simulink model "MotorSimlab4"  (R2015b)
settings: Solver=ode4  StartTime=0.0  StopTime=10  FixedStep=0.001  RelTol=1e-3
values from neighbouring files (symbols this model uses):
  Beq = BeqHigh    (= 0.015)    [transferfunctionlab4.m]
  Jeq = JeqPaper    (= 0.00213)    [transferfunctionlab4.m]
  Ka = KaHigh    (= 3420.59016393)    [transferfunctionlab4.m]
  Kb = KbHigh    (= 0.5376)    [transferfunctionlab4.m]
  Kg = KgHigh    (= 70)    [transferfunctionlab4.m]
  Rm = 2.6    [transferfunctionlab4.m]
undefined symbols (not defined in the file or in its folder): HIL, qc_get_step_size
libraries: quarc_library x4
settings Model: SimulationMode=external  ExtModeTrigDuration=10000  Creator=dilsizk  LastModifiedBy=dilsizk
settings SolverCC: PositivePriorityOrder=on
settings RTWCC: SystemTargetFile=quarc_win64.tlc  TemplateMakefile=quarc_default_tmf  Description=QUARC Win64 Target
settings STFCustomTargetCC: TargetPreCompLibLocation=C:\ProgramData\QUARC\lib\2015b\win64\release  GeneratePreprocessorConditionals=Use local settings  CPPClassGenCompliant=off
settings GRTTargetCC: TargetPreCompLibLocation=C:\ProgramData\QUARC\lib\2015b\win64\release  ParMdlRefBuildCompliant=off  CompOptLevelCompliant=off  CombineOutputUpdateFcns=off  MatFileLogging=off  CPPClassGenCompliant=off  GRTInterface=on  UseToolchainInfoCompliant=off  ExtMode=on  ExtModeMexFile=quarc_comm

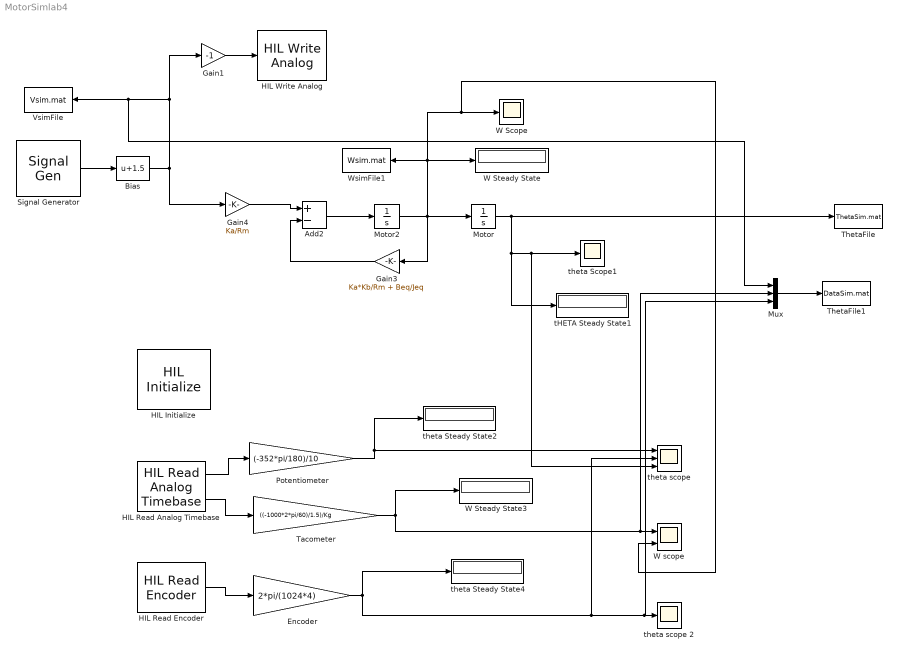
== system MotorSimlab4 ==
  Add2 : Sum  Inputs=+-
  Bias : Bias  Bias=1.5
  Encoder : Gain  Gain=2*pi/(1024*4)
  Gain1 : Gain  Gain=-1
  Gain3 : Gain  Gain=Ka*Kb/Rm + Beq/Jeq
  Gain4 : Gain  Gain=Ka/Rm
  HIL Initialize : quarc_library/Data Acquisition/Generic/Configuration/HIL Initialize  Priority=-99  object_name=HIL-2  board_type=q8_usb  board_number=0  board_options=update_rate=normal;decimation=1  exclusive=off  active=off  hardware_clocks=[0:2]  clock_modes=[]  initial_clock_frequencies=[]  set_clock_params_at_start=off  set_clock_params_at_switch_in=off  set_clock_frequencies_at_start=off  set_clock_frequencies_at_switch_in=off  analog_input_channels=[0:7]  analog_input_maximums=10  analog_input_minimums=-10  set_analog_input_params_at_start=on  set_analog_input_params_at_switch_in=off  analog_output_channels=[0:7]  analog_output_maximums=10  analog_output_minimums=-10  initial_analog_outputs=[0]  final_analog_outputs=[0]  watchdog_analog_outputs=0  set_analog_output_params_at_start=on  set_analog_output_params_at_switch_in=off  set_analog_outputs_at_start=on  set_analog_outputs_at_switch_in=off  set_analog_outputs_at_terminate=on  set_analog_outputs_at_switch_out=off  set_analog_outputs_on_watchdog=off  digital_input_channels=[]  digital_output_channels=[]  digital_output_configuration=[]  initial_digital_outputs=[1]  final_digital_outputs=[1]  watchdog_digital_outputs=[1]  set_digital_output_params_at_start=off  set_digital_output_params_at_switch_in=off  set_digital_outputs_at_start=on  set_digital_outputs_at_switch_in=off  set_digital_outputs_at_terminate=on  set_digital_outputs_at_switch_out=off  set_digital_outputs_on_watchdog=off  encoder_channels=[0:7]  quadrature=[4]  encoder_filter_frequency=[]  initial_encoder_counts=[0]  set_encoder_params_at_start=on  set_encoder_params_at_switch_in=off  set_encoder_counts_at_start=on  set_encoder_counts_at_switch_in=off  pwm_channels=[0:7]  pwm_modes=0  pwm_frequency=99.532799999999995e6/4095  pwm_configuration=[0]  pwm_alignment=[0]  pwm_polarity=[1]  pwm_leading_deadband=[0]  pwm_trailing_deadband=[0]  initial_pwm_outputs=[0]  final_pwm_outputs=[0]  watchdog_pwm_outputs=[0]  set_pwm_params_at_start=on  set_pwm_params_at_switch_in=off  set_pwm_outputs_at_start=on  set_pwm_outputs_at_switch_in=off  set_pwm_outputs_at_terminate=on  set_pwm_outputs_at_switch_out=off  set_pwm_outputs_on_watchdog=off  other_output_channels=[]  initial_other_outputs=[]  final_other_outputs=[]  watchdog_other_outputs=[]  set_other_outputs_at_start=off  set_other_outputs_at_switch_in=off  set_other_outputs_at_terminate=off  set_other_outputs_at_switch_out=off  set_other_outputs_on_watchdog=off
  HIL Read Analog Timebase : quarc_library/Data Acquisition/Generic/Timebases/HIL Read Analog Timebase  object_name=HIL-2  clock=0  channels=[0:1]  samples_in_buffer=max(ceil(1/qc_get_step_size), 1)  active=on  vector_output=off
      settings: AttributesFormatString=(%<object_name>)
  HIL Read Encoder : quarc_library/Data Acquisition/Generic/Immediate I//O/HIL Read Encoder  object_name=HIL-2  channels=[0]  sample_time=qc_get_step_size  active=on  vector_output=off  data_type_mode=Inherit via back propagation  data_type=double
  HIL Write Analog : quarc_library/Data Acquisition/Generic/Immediate I//O/HIL Write Analog  object_name=HIL-2  channels=0  sample_time=-1  active=off  vector_input=off
  Motor : Integrator
  Motor2 : Integrator
  Mux : Mux  Inputs=3
  Potentiometer : Gain  Gain=(-352*pi/180)/10
  Signal Generator : SignalGenerator  WaveForm=square  Frequency=0.4
  Tacometer : Gain  Gain=((-1000*2*pi/60)/1.5)/Kg
  ThetaFile : ToFile  Filename=ThetaSim.mat  MatrixName=Tdata
  ThetaFile1 : ToFile  Filename=DataSim.mat  MatrixName=data
  VsimFile : ToFile  Filename=Vsim.mat  MatrixName=Vdata
  W Steady State : Display
  W Steady State3 : Display
  W Scope : Scope
  W scope : Scope  NumInputPorts=2
  WsimFile1 : ToFile  Filename=Wsim.mat  MatrixName=Wdata
  tHETA Steady State1 : Display
  theta Steady State2 : Display
  theta Steady State4 : Display
  theta Scope1 : Scope
  theta scope : Scope  NumInputPorts=3
  theta scope 2 : Scope
  wires:
  Bias/1 -> Gain4/1, Gain1/1, Mux/1, VsimFile/1
  Gain4/1 -> Add2/1
  Add2/1 -> Motor2/1
  Gain3/1 -> Add2/2
  Motor2/1 -> Motor/1, Gain3/1, W Steady State/1, WsimFile1/1, W scope/2, W Scope/1
  Motor/1 -> tHETA Steady State1/1, theta scope/3, theta Scope1/1, ThetaFile/1
  Gain1/1 -> HIL Write Analog/1
  HIL Read Encoder/1 -> Encoder/1
  Potentiometer/1 -> theta Steady State2/1, theta scope/1
  HIL Read Analog Timebase/2 -> Tacometer/1
  HIL Read Analog Timebase/1 -> Potentiometer/1
  Tacometer/1 -> W Steady State3/1, Mux/2, W scope/1
  Encoder/1 -> theta Steady State4/1, Mux/3, theta scope 2/1, theta scope/2
  Signal Generator/1 -> Bias/1
  Mux/1 -> ThetaFile1/1
